simulink model "lynchpark_forcecontrol_v1b"  (R2022b)
settings: Solver=FixedStepDiscrete  StartTime=0.0  StopTime=Inf  FixedStep=0.001  RelTol=1e-3  EnableMultiTasking=on
PreLoadFcn:
  | set_param(gcs, 'RTWSystemTargetFile', 'franka_emika_panda.tlc');
  | % demos_common_configs();
values from neighbouring files (symbols this model uses):
  init_delay = 10    [lynchpark_forcecontrol_v1_init.m]
  q_init = [65*pi/128, 59*pi/512, 0, -315 * pi/512, 0, 48*pi/64, 14*pi/64]    [lynchpark_forcecontrol_v1_init.m]
  V_damp = diag([10 10 10 10 10 10])    [lynchpark_forcecontrol_v1_init.m]
undefined symbols (not defined in the file or in its folder): DiscIntNeverNeededParam, FR_EE_LC, R_O_LC
libraries: spsSampleandHoldLib x18, franka_simulink_library x7, simulink x2, etargetslib x2, dspnetwork x2, dspsigops x1
settings Model: SimulationMode=external  ExtModeTrigDuration=10000  Creator=vasi_ko  LastModifiedBy=host
settings SolverCC: AlgebraicLoopSolver=TrustRegion
settings DataIOCC: LimitDataPoints=on  SaveFormat=Array  ReturnWorkspaceOutputs=off
settings OptimizationCC: EnhancedBackFolding=on  PassReuseOutputArgsThreshold=0  OptimizeBlockOrder=speed  DifferentSizesBufferReuse=on  OptimizationCustomize=off
settings DebuggingCC: SolverPrmCheckMsg=warning  ParameterTunabilityLossMsg=error  UnconnectedInputMsg=warning  UnconnectedOutputMsg=warning  UnconnectedLineMsg=warning  SFUnexpectedBacktrackingDiag=warning  SFNoUnconditionalDefaultTransitionDiag=warning  SFExecutionAtInitializationDiag=none  SFMachineParentedDataDiag=warning  ArithmeticOperatorsInVariantConditions=warning
settings HardwareCC: ProdBitPerLong=64  ProdHWDeviceType=Intel->x86-64 (Linux 64)
settings ModelReferenceCC: EnableRefExpFcnMdlSchedulingChecks=on  PropagateSignalLabelsOutOfModel=off
settings SFSimCC: SimUseLocalCustomCode=off  MATLABDynamicMemAlloc=off  CustomCodeUndefinedFunction=UseInterfaceOnly  SimTargetLang=C++
settings RTWCC: SystemTargetFile=franka_emika_panda.tlc  RTWVerbose=off  RTWUseLocalCustomCode=off  Toolchain=Franka Simulink | gmake (64-bit linux)  BuildConfiguration=Faster Runs  TargetLang=C++  DLArmComputeVersion=19.05
settings CodeAppCC: ForceParamTrailComments=on  OperatorAnnotations=on
settings STFCustomTargetCC: TargetLangStandard=C99 (ISO)  ModelReferenceCompliant=off  MatFileLogging=on  GRTInterface=on  UseToolchainInfoCompliant=on  SystemTargetFile=franka_emika_panda.tlc
settings GRTTargetCC: ModelReferenceCompliant=off  ParMdlRefBuildCompliant=off  CompOptLevelCompliant=off  ConcurrentExecutionCompliant=off  CombineOutputUpdateFcns=off  CPPClassGenCompliant=off  GRTInterface=on  ExtModeStaticAlloc=on  ExtModeTransport=1  ExtModeMexFile=ext_xcp  ExtModeIntrfLevel=Level2 - Open
settings ConfigComp: CovMetricSettings=dw  CovSaveCumulativeToWorkspaceVar=on  CovSaveSingleToWorkspaceVar=on  CovExternalEMLEnable=off  CovSFcnEnable=off

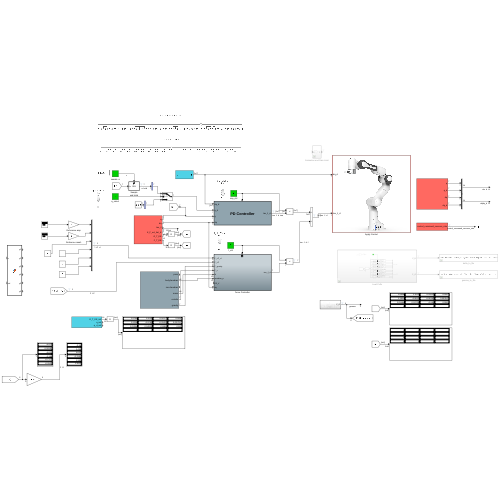
[thumbnail: Simulink's stored preview of the top-level diagram]
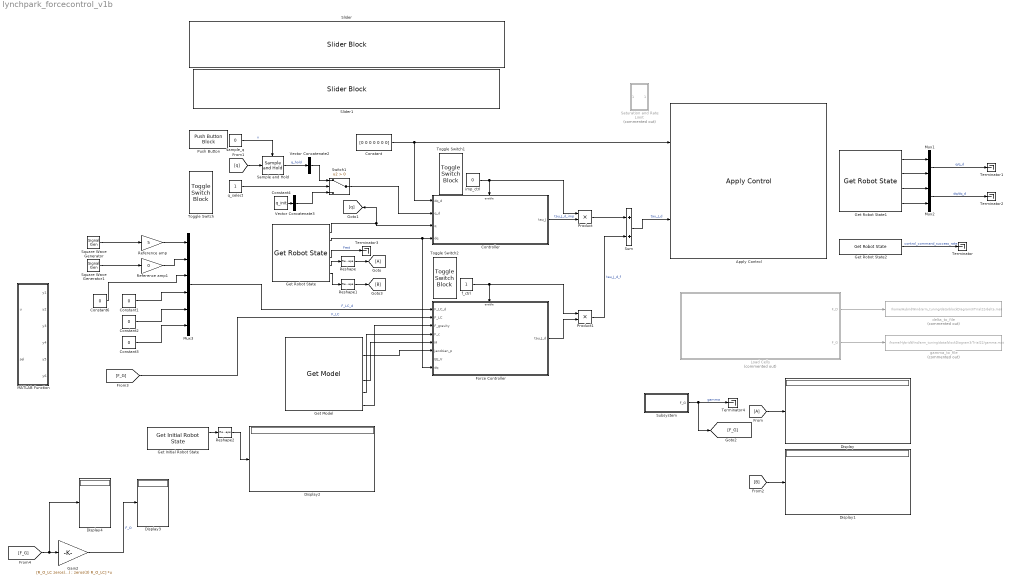
== system lynchpark_forcecontrol_v1b ==
  Apply Control : franka_simulink_library/Apply Control  robot_ip=robot_ip  gripper_attached=off  control_mode=Torque Control - Joint Velocities  controller_choice=Joint Impedance Controller  elbow_control=on  collision_thresholds=100*ones(1,52)  joint_impedance=joint_impedance  cartesian_impedance=cartesian_impedance  load_inertia=load_inertia  EE_T_K=EE_T_K  init_joint_configuration_req=off  init_joint_configuration=q_init
      settings: SourceProductName=Franka Emika Simulink Support Package
  Constant : Constant  Value=[0 0 0 0 0 0 0]  VectorParams1D=off
  Constant{1..3,6} (4 alike) : Constant  Value=0
  Constant4 : Constant  Value=q_init
  Controller : Subsystem
      mask Display:
      | % pos = get_param(gcb, 'Position');
      | 
      | disp('{\bf\fontsize{18}PD Controller}', 'texmode','on');
      | 
      | block_icon('Controller')
      | 
      | port_label('output',1,'tau_J_d');
      | 
      | port_label('input',2,'q_d');
      | port_label('input',1,'dq_d');
      | port_label('input',3,'q');
      | port_label('input',4,'dq');
  Display{,1..4} (5 alike) : Display
  "Force Controller " : Subsystem
  From : From
  Gain2 : Gain  Gain=[R_O_LC zeros(3) ; zeros(3) R_O_LC]  Multiplication=Matrix(K*u)
  Get Initial Robot State : franka_simulink_library/Get Initial Robot State  robot_ip=robot_ip  signals_requested='O_T_EE q q_d'
      settings: SourceProductName=Franka Emika Simulink Support Package
  Get Model : franka_simulink_library/Get Model  robot_ip=robot_ip
      settings: SourceProductName=Franka Emika Simulink Support Package
  Get Robot State : franka_simulink_library/Get Robot State  robot_ip=robot_ip  signals_requested='q dq tau_J K_F_ext_hat_K O_T_EE F_T_EE'
      settings: SourceProductName=Franka Emika Simulink Support Package
  Get Robot State1 : franka_simulink_library/Get Robot State  robot_ip=robot_ip  signals_requested='q q_d dq dq_d'
      settings: SourceProductName=Franka Emika Simulink Support Package
  Get Robot State2 : franka_simulink_library/Get Robot State  robot_ip=robot_ip  signals_requested='control_command_success_rate'
      settings: SourceProductName=Franka Emika Simulink Support Package
  Goto : Goto
  Load Cells : Subsystem  Commented=on
  MATLAB Function : MATLAB Function  TreatAsAtomicUnit=on
  Mux1 : Mux  Inputs=2
  Mux2 : Mux  Inputs=2
  Mux3 : Mux  Inputs=6
  Product : Product
  Product1 : Product
  Push Button : PushButtonBlock  OffValue=0.000000
  Reference amp : Gain  Gain=5
  Reference amp1 : Gain  Gain=0
  Reshape : Reshape  OutputDimensionality=Customize  OutputDimensions=[4,4]
  Reshape1 : Reshape  OutputDimensionality=Customize  OutputDimensions=[4,4]
  Reshape2 : Reshape  OutputDimensionality=Customize  OutputDimensions=[4,4]
  Sample and Hold : dspsigops/Sample and Hold  trig=Rising edge  initCond=q_init  latchinput=off
  Saturation and Rate Limit : Subsystem  Commented=on
  Slider : SliderBlock  ScaleMax=7  TickInterval=0.25
  Slider1 : SliderBlock  ScaleMax=2
  Square Wave Generator : SignalGenerator  WaveForm=square  Frequency=1/10
  Square Wave Generator1 : SignalGenerator  WaveForm=square  Frequency=1/10
  Subsystem : Subsystem
  Sum : Sum
  Switch1 : Switch  Criteria=u2 > Threshold  SaturateOnIntegerOverflow=off  InputSameDT=off
  Terminator{,1..4} (5 alike) : Terminator
  Toggle Switch : ToggleSwitchBlock
      settings: Values={{'Off', 'On'}, [0 1]}
  Toggle Switch1 : ToggleSwitchBlock
      settings: Values={{'Off', 'On'}, [0 1]}
  Toggle Switch2 : ToggleSwitchBlock
      settings: Values={{'Off', 'On'}, [0 1]}
  Vector Concatenate2 : Concatenate  NumInputs=1
  Vector Concatenate3 : Concatenate  NumInputs=1
  delta_to_file : ToFile  Commented=on  Filename=/home/HybridWind/arm_tuning/data/blockDiagram3/Trial22/delta.mat  MatrixName=delta
  f_ctrl : Constant
  gamma_to_file : ToFile  Commented=on  Filename=/home/HybridWind/arm_tuning/data/blockDiagram3/Trial22/gamma.mat  MatrixName=gamma
  imp_ctrl : Constant  Value=0
  q_select : Constant
  sample_q : Constant  Value=0
  wires:
  Switch1/1 -> Controller/2(q_d)
  Get Robot State1/2 -> Mux1/2
  f_ctrl/1 -> Product1/1, "Force Controller "/Enable
  Vector Concatenate2/1 -> Switch1/1
  Load Cells/1(F_D) -> delta_to_file/1
  Get Robot State/1 -> Controller/3(q), [q]
  Mux1/1 -> Terminator1/1  "q/q_d"
  Get Robot State1/3 -> Mux2/1
  [q] -> Sample and Hold/1
  Get Robot State1/1 -> Mux1/1
  Get Model/4 -> "Force Controller "/5(M)
  imp_ctrl/1 -> Product/1, Controller/Enable
  Get Model/5 -> "Force Controller "/4(F_c)
  Get Robot State/2 -> "Force Controller "/8(dq), Controller/4(dq)
  Constant4/1 -> Vector Concatenate3/1
  Get Robot State1/4 -> Mux2/2
  "Force Controller "/1(tau_J_d) -> Product1/2
  sample_q/1 -> Sample and Hold/Trigger  "x"
  Sample and Hold/1 -> Vector Concatenate2/1  "q_hold"
  Get Model/6 -> "Force Controller "/3(F_gravity)
  q_select/1 -> Switch1/2
  Sum/1 -> Apply Control/2  "tau_J_d"
  Mux2/1 -> Terminator2/1  "dq/dq_d"
  Product/1 -> Sum/1
  Vector Concatenate3/1 -> Switch1/3
  Load Cells/2(F_G) -> gamma_to_file/1
  Controller/1(tau_J) -> Product/2  "tau_J_d_imp"
  Get Robot State2/1 -> Terminator/1  "control_command_success_rate"
  Product1/1 -> Sum/2  "tau_J_d_f"
  Constant/1 -> Apply Control/1, Controller/1(dq_d)
  Get Robot State/4 -> Terminator3/1  "Fest"
  Get Robot State/5 -> Reshape/1
  From/1 -> Display/1
  Reshape/1 -> Goto/1
  Reshape1/1 -> [B]
  Get Robot State/6 -> Reshape1/1
  [B] -> Display1/1
  Get Initial Robot State/1 -> Reshape2/1
  Reshape2/1 -> Display2/1
  Subsystem/1(F_G) -> [F_G], Terminator4/1  "gamma"
  [F_G] -> "Force Controller "/2(F_LC)  "F_LC"
  Mux3/1 -> "Force Controller "/1(F_LC_d)  "F_LC_d"
  Reference amp/1 -> Mux3/1
  Constant1/1 -> Mux3/4
  Reference amp1/1 -> Mux3/2
  Constant2/1 -> Mux3/5
  Constant3/1 -> Mux3/6
  Square Wave Generator/1 -> Reference amp/1
  Constant6/1 -> Mux3/3
  [F_G] -> Display4/1, Gain2/1
  Gain2/1 -> Display3/1  "F_O"
  Square Wave Generator1/1 -> Reference amp1/1
  Get Model/2 -> "Force Controller "/6(jacobian_p)

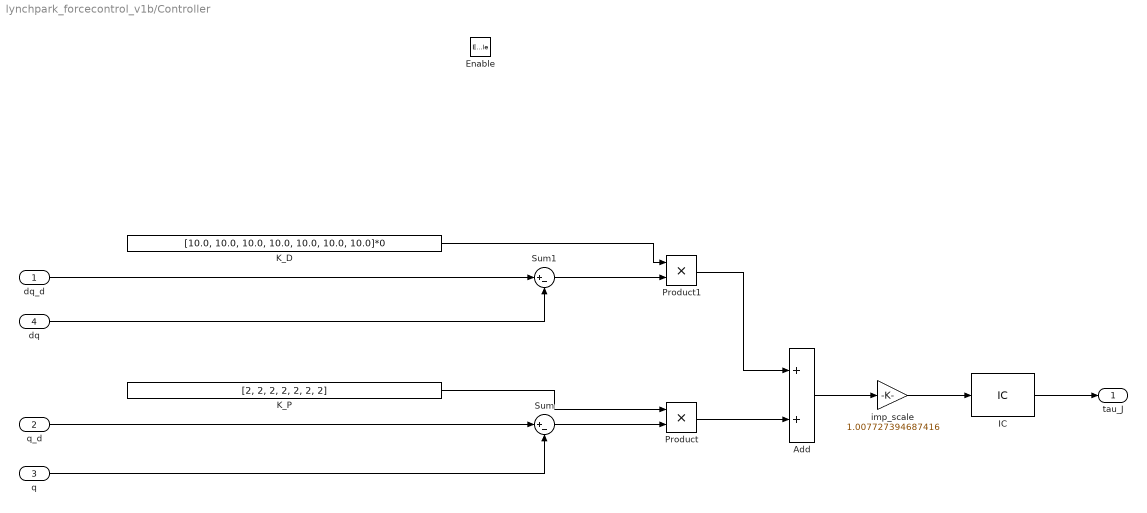
== system lynchpark_forcecontrol_v1b/Controller ==
  dq_d : Inport
  q_d : Inport  Port=2
  q : Inport  Port=3
  dq : Inport  Port=4
  Enable : EnablePort  StatesWhenEnabling=reset
  Add : Sum
  IC : InitialCondition  Value=zeros(1,7)
  K_D : Constant  Value=[10.0, 10.0, 10.0, 10.0, 10.0, 10.0, 10.0]*0  VectorParams1D=off  SampleTime=-1
  K_P : Constant  Value=[2, 2, 2, 2, 2, 2, 2]  VectorParams1D=off  SampleTime=-1
  Product : Product
  Product1 : Product
  Sum : Sum  Inputs=|+-
  Sum1 : Sum  Inputs=|+-
  imp_scale : Gain  Gain=1.007727394687416
  tau_J : Outport  VectorParamsAs1DForOutWhenUnconnected=off
  wires:
  Add/1 -> imp_scale/1
  Sum1/1 -> Product1/2
  dq/1 -> Sum1/2
  q_d/1 -> Sum/1
  dq_d/1 -> Sum1/1
  Product1/1 -> Add/1
  Product/1 -> Add/2
  Sum/1 -> Product/2
  q/1 -> Sum/2
  K_P/1 -> Product/1
  K_D/1 -> Product1/1
  IC/1 -> tau_J/1
  imp_scale/1 -> IC/1

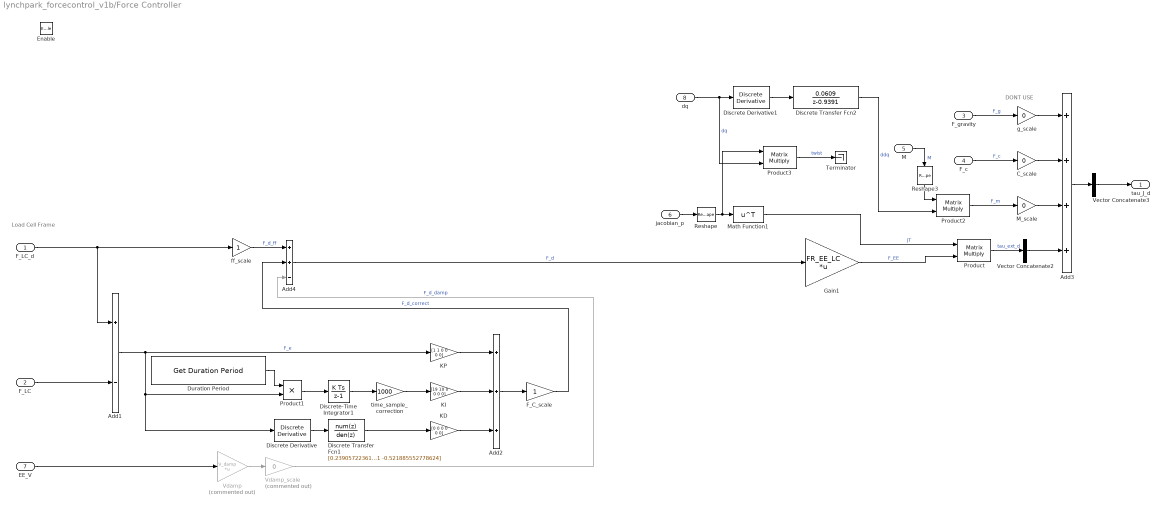
== system lynchpark_forcecontrol_v1b/Force Controller  ==
  note: DONT USE
  note: Load Cell Frame
  F_LC_d : Inport
  F_LC : Inport  Port=2
  F_gravity : Inport  Port=3
  F_c : Inport  Port=4
  M : Inport  Port=5
  jacobian_p : Inport  Port=6
  EE_V : Inport  Port=7
  dq : Inport  Port=8
  Enable : EnablePort  StatesWhenEnabling=reset
  Add1 : Sum  Inputs=+-
  Add2 : Sum  Inputs=+++
  Add3 : Sum  Inputs=++++
  Add4 : Sum  Inputs=++-
  C_scale : Gain  Gain=0
  Discrete Transfer Fcn1 : DiscreteTransferFcn  Numerator=[0.239057223610688 0.239057223610688]  Denominator=[1 -0.521885552778624]
  Discrete Transfer Fcn2 : DiscreteTransferFcn  Numerator=[0.0609]  Denominator=[1 -0.9391]
  Discrete Derivative : simulink/Discrete/Discrete Derivative  gainval=1.0  ICPrevScaledInput=0.0  OutMin=[]  OutMax=[]  OutDataType=fixdt(1, 16)  OutScaling=2^-10  DoSatur=off
  Discrete Derivative1 : simulink/Discrete/Discrete Derivative  gainval=1.0  ICPrevScaledInput=0.0  OutMin=[]  OutMax=[]  OutDataType=fixdt(1, 16)  OutScaling=2^-10  DoSatur=off
  Discrete-Time Integrator1 : DiscreteIntegrator  SampleTime=0.001  ICPrevOutput=DiscIntNeverNeededParam  ICPrevScaledInput=DiscIntNeverNeededParam
  Duration Period : franka_simulink_library/Get Duration Period  robot_ip=robot_ip
      settings: SourceProductName=Franka Emika Simulink Support Package
  F_C_scale : Gain
  Gain1 : Gain  Gain=FR_EE_LC  Multiplication=Matrix(K*u)
  KD : Gain  Gain=[0 0 0 0 0 0]
  KI : Gain  Gain=[19 10 0 0 0 0]
  KP : Gain  Gain=[1 1 0 0 0 0]
  M_scale : Gain  Gain=0
  Math Function1 : Math  Operator=transpose  SignedPower=on
  Product : Product  Multiplication=Matrix(*)
  Product1 : Product
  Product2 : Product  Multiplication=Matrix(*)
  Product3 : Product  Multiplication=Matrix(*)
  Reshape : Reshape  OutputDimensionality=Customize  OutputDimensions=[6,7]
  Reshape3 : Reshape  OutputDimensionality=Customize  OutputDimensions=[7,7]
  Terminator : Terminator
  Vdamp : Gain  Commented=on  Gain=V_damp  Multiplication=Matrix(K*u)
  Vdamp_scale : Gain  Commented=on  Gain=0
  Vector Concatenate2 : Concatenate  NumInputs=1
  Vector Concatenate3 : Concatenate  NumInputs=1
  ff_scale : Gain
  g_scale : Gain  Gain=0
  time_sample_correction : Gain  Gain=1000
  tau_J_d : Outport  InitialOutput=[0 0 0 0 0 0 0]  VectorParamsAs1DForOutWhenUnconnected=off
  wires:
  Add1/1 -> KP/1, Discrete Derivative/1, Product1/2  "F_e"
  Discrete Transfer Fcn1/1 -> KD/1
  KD/1 -> Add2/3
  KP/1 -> Add2/1
  F_gravity/1 -> g_scale/1  "F_g"
  KI/1 -> Add2/2
  Duration Period/1 -> Product1/1
  Discrete Derivative/1 -> Discrete Transfer Fcn1/1
  Product1/1 -> Discrete-Time Integrator1/1
  Discrete-Time Integrator1/1 -> time_sample_correction/1
  time_sample_correction/1 -> KI/1
  F_c/1 -> C_scale/1  "F_c"
  Product2/1 -> M_scale/1  "F_m"
  g_scale/1 -> Add3/1
  Reshape/1 -> Product3/1, Math Function1/1
  jacobian_p/1 -> Reshape/1
  Math Function1/1 -> Product/1  "JT"
  Product/1 -> Vector Concatenate2/1  "tau_ext_d"
  F_LC/1 -> Add1/2
  Add3/1 -> Vector Concatenate3/1
  ff_scale/1 -> Add4/1  "F_d_ff"
  Add4/1 -> Gain1/1  "F_d"
  Add2/1 -> F_C_scale/1
  Vdamp/1 -> Vdamp_scale/1
  EE_V/1 -> Vdamp/1
  Vdamp_scale/1 -> Add4/3  "F_d_damp"
  F_C_scale/1 -> Add4/2  "F_d_correct"
  C_scale/1 -> Add3/2
  M_scale/1 -> Add3/3
  M/1 -> Reshape3/1  "M"
  Discrete Transfer Fcn2/1 -> Product2/2  "ddq"
  Discrete Derivative1/1 -> Discrete Transfer Fcn2/1
  dq/1 -> Discrete Derivative1/1, Product3/2  "dq"
  Product3/1 -> Terminator/1  "twist"
  Vector Concatenate3/1 -> tau_J_d/1
  Vector Concatenate2/1 -> Add3/4
  Reshape3/1 -> Product2/1
  F_LC_d/1 -> Add1/1, ff_scale/1
  Gain1/1 -> Product/2  "F_EE"

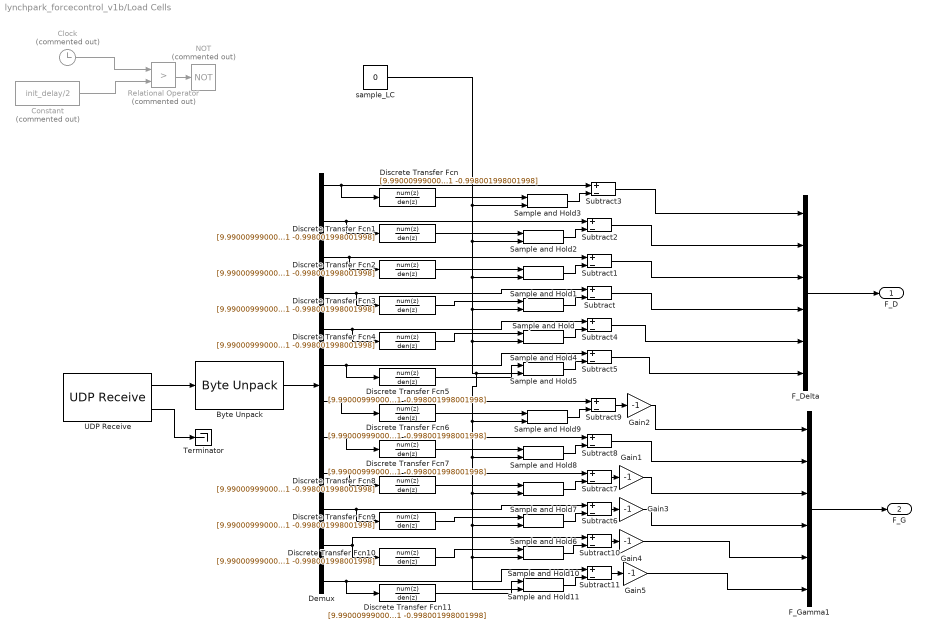
== system lynchpark_forcecontrol_v1b/Load Cells ==
  Byte Unpack : etargetslib/Byte Unpack  dimensions={[12]}  datatypes={'double'}  byteAlign=1
  Clock : Clock  Commented=on
  Constant : Constant  Commented=on  Value=init_delay/2
  Demux : Demux  Outputs=12
  Discrete Transfer Fcn{,1..11} (12 alike) : DiscreteTransferFcn  Numerator=[9.990009990009990e-04 9.990009990009990e-04]  Denominator=[1 -0.998001998001998]
  F_Delta : Mux  Inputs=6
  F_Gamma1 : Mux  Inputs=6
  Gain{1..5} (5 alike) : Gain  Gain=-1
  NOT : Logic  Commented=on  Operator=NOT  IconShape=distinctive  AllPortsSameDT=off  OutDataTypeStr=boolean
  Relational Operator : RelationalOperator  Commented=on  Operator=>  OutDataTypeStr=boolean  RndMeth=Simplest  InputSameDT=off
  Sample and Hold{,1..11} (12 alike) : spsSampleandHoldLib/Sample and Hold  ic=0  Ts=0
  Subtract{,1..11} (12 alike) : Sum  Inputs=+-
  Terminator : Terminator
  UDP Receive : dspnetwork/UDP Receive  localURL='0.0.0.0'  localPort=8002  remoteURL='10.10.10.15'  remotePort=-1  recvBufferSize=8192  dims=96  signalDatatype=uint8  isComplex=off  isVarSize=off  showBlockingTime=on  blockingTime=inf  sampletime=0.001  blockPlatform=HOST
  sample_LC : Constant  Value=0
  F_D : Outport
  F_G : Outport  Port=2
  wires:
  UDP Receive/1 -> Byte Unpack/1
  Constant/1 -> Relational Operator/2
  Relational Operator/1 -> NOT/1
  Sample and Hold/1 -> Subtract/2
  UDP Receive/2 -> Terminator/1
  Demux/4 -> Discrete Transfer Fcn3/1, Subtract/1
  Clock/1 -> Relational Operator/1
  Byte Unpack/1 -> Demux/1
  Demux/3 -> Discrete Transfer Fcn2/1, Subtract1/1
  Sample and Hold1/1 -> Subtract1/2
  Subtract1/1 -> F_Delta/3
  Subtract2/1 -> F_Delta/2
  Sample and Hold2/1 -> Subtract2/2
  Demux/2 -> Discrete Transfer Fcn1/1, Subtract2/1
  Sample and Hold3/1 -> Subtract3/2
  Subtract4/1 -> F_Delta/5
  Sample and Hold4/1 -> Subtract4/2
  Demux/5 -> Discrete Transfer Fcn4/1, Subtract4/1
  Demux/6 -> Discrete Transfer Fcn5/1, Subtract5/1
  Sample and Hold5/1 -> Subtract5/2
  Subtract5/1 -> F_Delta/6
  Subtract3/1 -> F_Delta/1
  Subtract/1 -> F_Delta/4
  F_Delta/1 -> F_D/1
  Demux/1 -> Discrete Transfer Fcn/1, Subtract3/1
  Discrete Transfer Fcn/1 -> Sample and Hold3/1
  Discrete Transfer Fcn1/1 -> Sample and Hold2/1
  Discrete Transfer Fcn2/1 -> Sample and Hold1/1
  Discrete Transfer Fcn3/1 -> Sample and Hold/1
  Discrete Transfer Fcn4/1 -> Sample and Hold4/1
  Discrete Transfer Fcn5/1 -> Sample and Hold5/1
  Discrete Transfer Fcn11/1 -> Sample and Hold11/1
  Discrete Transfer Fcn10/1 -> Sample and Hold10/1
  Discrete Transfer Fcn9/1 -> Sample and Hold6/1
  Discrete Transfer Fcn8/1 -> Sample and Hold7/1
  Discrete Transfer Fcn7/1 -> Sample and Hold8/1
  Discrete Transfer Fcn6/1 -> Sample and Hold9/1
  Demux/7 -> Subtract9/1, Discrete Transfer Fcn6/1
  F_Gamma1/1 -> F_G/1
  Gain3/1 -> F_Gamma1/4
  Gain2/1 -> F_Gamma1/1
  Subtract11/1 -> Gain5/1
  Sample and Hold11/1 -> Subtract11/2
  sample_LC/1 -> Sample and Hold3/2, Sample and Hold2/2, Sample and Hold1/2, Sample and Hold6/2, Sample and Hold10/2, Sample and Hold11/2, Sample and Hold7/2, Sample and Hold8/2, Sample and Hold9/2, Sample and Hold5/2, Sample and Hold4/2, Sample and Hold/2
  Demux/12 -> Subtract11/1, Discrete Transfer Fcn11/1
  Demux/11 -> Subtract10/1, Discrete Transfer Fcn10/1
  Sample and Hold10/1 -> Subtract10/2
  Gain4/1 -> F_Gamma1/5
  Subtract9/1 -> Gain2/1
  Sample and Hold9/1 -> Subtract9/2
  Demux/8 -> Subtract8/1, Discrete Transfer Fcn7/1
  Sample and Hold8/1 -> Subtract8/2
  Subtract8/1 -> F_Gamma1/2
  Gain1/1 -> F_Gamma1/3
  Sample and Hold7/1 -> Subtract7/2
  Demux/9 -> Subtract7/1, Discrete Transfer Fcn8/1
  Demux/10 -> Subtract6/1, Discrete Transfer Fcn9/1
  Sample and Hold6/1 -> Subtract6/2
  Subtract6/1 -> Gain3/1
  Subtract7/1 -> Gain1/1
  Subtract10/1 -> Gain4/1
  Gain5/1 -> F_Gamma1/6

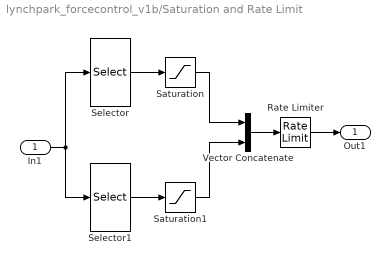
== system lynchpark_forcecontrol_v1b/Saturation and Rate Limit ==
  In1 : Inport
  Rate Limiter : RateLimiter  RisingSlewLimit=1000  FallingSlewLimit=-1000  SampleTimeMode=inherited
  Saturation : Saturate  UpperLimit=87  LowerLimit=-87
  Saturation1 : Saturate  UpperLimit=12  LowerLimit=-12
  Selector : Selector  InputPortWidth=7  IndexOptions=Index vector (dialog)  Indices=[1 2 3 4]  OutputSizes=1
  Selector1 : Selector  InputPortWidth=7  IndexOptions=Index vector (dialog)  Indices=[5 6 7]  OutputSizes=1
  Vector Concatenate : Concatenate
  Out1 : Outport
  wires:
  Saturation1/1 -> Vector Concatenate/2
  Vector Concatenate/1 -> Rate Limiter/1
  Saturation/1 -> Vector Concatenate/1
  Rate Limiter/1 -> Out1/1
  Selector1/1 -> Saturation1/1
  Selector/1 -> Saturation/1
  In1/1 -> Selector1/1, Selector/1

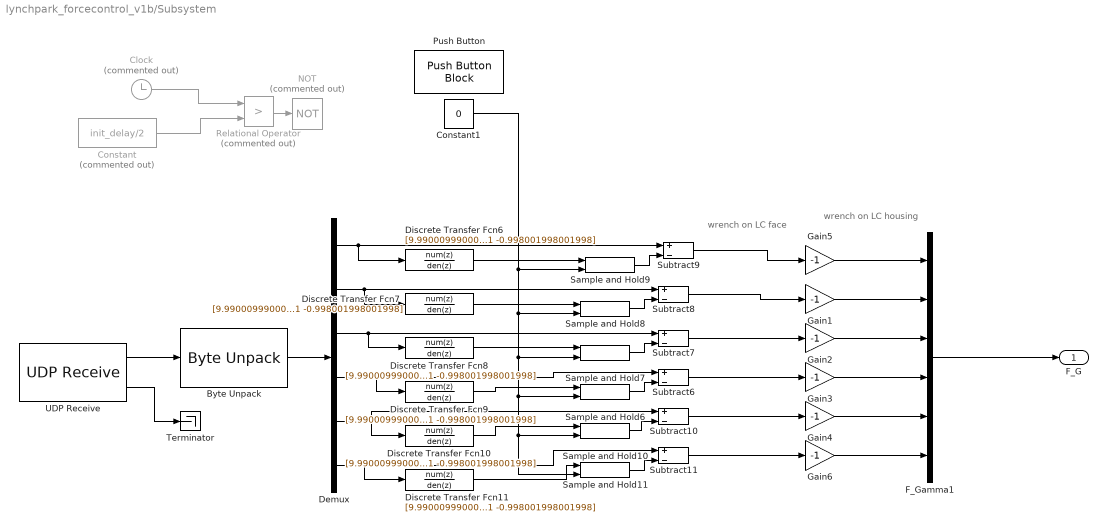
== system lynchpark_forcecontrol_v1b/Subsystem ==
  note: wrench on LC face
  note: wrench on LC housing
  Byte Unpack : etargetslib/Byte Unpack  dimensions={[6]}  datatypes={'double'}  byteAlign=1
  Clock : Clock  Commented=on
  Constant : Constant  Commented=on  Value=init_delay/2
  Constant1 : Constant  Value=0
  Demux : Demux  Outputs=6
  Discrete Transfer Fcn{6..11} (6 alike) : DiscreteTransferFcn  Numerator=[9.990009990009990e-04 9.990009990009990e-04]  Denominator=[1 -0.998001998001998]
  F_Gamma1 : Mux  Inputs=6
  Gain{1..6} (6 alike) : Gain  Gain=-1
  NOT : Logic  Commented=on  Operator=NOT  IconShape=distinctive  AllPortsSameDT=off  OutDataTypeStr=boolean
  Push Button : PushButtonBlock  OffValue=0.000000
  Relational Operator : RelationalOperator  Commented=on  Operator=>  OutDataTypeStr=boolean  RndMeth=Simplest  InputSameDT=off
  Sample and Hold{6..11} (6 alike) : spsSampleandHoldLib/Sample and Hold  ic=0  Ts=0
  Subtract{6..11} (6 alike) : Sum  Inputs=+-
  Terminator : Terminator
  UDP Receive : dspnetwork/UDP Receive  localURL='0.0.0.0'  localPort=8002  remoteURL='10.10.10.15'  remotePort=-1  recvBufferSize=8192  dims=96/2  signalDatatype=uint8  isComplex=off  isVarSize=off  showBlockingTime=on  blockingTime=inf  sampletime=0.001  blockPlatform=HOST
  F_G : Outport
  wires:
  Subtract10/1 -> Gain4/1
  Sample and Hold7/1 -> Subtract7/2
  Discrete Transfer Fcn7/1 -> Sample and Hold8/1
  Demux/2 -> Subtract8/1, Discrete Transfer Fcn7/1
  Subtract7/1 -> Gain2/1
  Sample and Hold8/1 -> Subtract8/2
  Demux/6 -> Subtract11/1, Discrete Transfer Fcn11/1
  Demux/1 -> Subtract9/1, Discrete Transfer Fcn6/1
  Demux/4 -> Subtract6/1, Discrete Transfer Fcn9/1
  Constant1/1 -> Sample and Hold6/2, Sample and Hold10/2, Sample and Hold11/2, Sample and Hold7/2, Sample and Hold8/2, Sample and Hold9/2
  Subtract9/1 -> Gain5/1
  Discrete Transfer Fcn9/1 -> Sample and Hold6/1
  Sample and Hold9/1 -> Subtract9/2
  Subtract8/1 -> Gain1/1
  Sample and Hold11/1 -> Subtract11/2
  Demux/3 -> Subtract7/1, Discrete Transfer Fcn8/1
  Sample and Hold10/1 -> Subtract10/2
  Sample and Hold6/1 -> Subtract6/2
  Demux/5 -> Subtract10/1, Discrete Transfer Fcn10/1
  Subtract11/1 -> Gain6/1
  Discrete Transfer Fcn8/1 -> Sample and Hold7/1
  Subtract6/1 -> Gain3/1
  Discrete Transfer Fcn11/1 -> Sample and Hold11/1
  Discrete Transfer Fcn6/1 -> Sample and Hold9/1
  Discrete Transfer Fcn10/1 -> Sample and Hold10/1
  UDP Receive/1 -> Byte Unpack/1
  Byte Unpack/1 -> Demux/1
  UDP Receive/2 -> Terminator/1
  Clock/1 -> Relational Operator/1
  Relational Operator/1 -> NOT/1
  Constant/1 -> Relational Operator/2
  F_Gamma1/1 -> F_G/1
  Gain5/1 -> F_Gamma1/1
  Gain1/1 -> F_Gamma1/2
  Gain2/1 -> F_Gamma1/3
  Gain3/1 -> F_Gamma1/4
  Gain4/1 -> F_Gamma1/5
  Gain6/1 -> F_Gamma1/6

== matlab function lynchpark_forcecontrol_v1b/MATLAB Function ==
  data: u input; y1 output; sel input; y2 output; y3 output; y4 output; y5 output; y6 output
function [y1, y2, y3, y4, y5, y6] = fcn(u, sel)

y1 = 0;
y2 = 0;
y3 = 0;
y4 = 0;
y5 = 0;
y6 = 0;

switch sel
    case 1
        y1 = u;
    case 2
        y2 = u;
    case 3
        y3 = u;
    case 4
        y4 = u;
    case 5
        y5 = u;
    case 6
        y6 = u;
    otherwise
        y1 = 0;
end
